simulink model "kalman_test"  (R2016b)
settings: Solver=VariableStepAuto  StartTime=0.0  StopTime=10  RelTol=1e-3
settings Model: Creator=Anass  LastModifiedBy=Anass

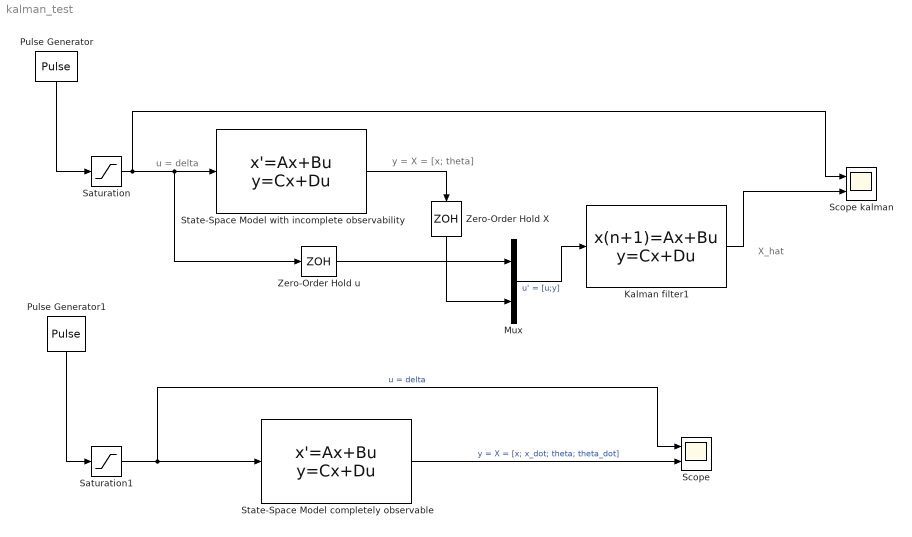
== system kalman_test ==
  note: X_hat
  note: y = X = [x; theta]
  note: u = delta
  Kalman filter1 : DiscreteStateSpace  A=|  B=|  C=eye(4)  D=zeros(4,3)  X0=[1;0;pi;0]  SampleTime=0.01  StateIdentifier=X_hat
      A=|
      | [    0.9697    0.0100   -0.0012         0;
      |    -0.0460    0.8959   -0.0171         0;
      |    -0.0012         0    0.9939    0.0100;
      |     0.0129   -0.0431   -0.3693    0.9938]
      B=|
      | [         0    0.0303    0.0012;
      |     0.5129    0.0460    0.0171;
      |          0    0.0012    0.0061;
      |     0.2102   -0.0129    0.0019]
  Mux : Mux  Inputs=2
  Pulse Generator : DiscretePulseGenerator  PulseType=Time based  Amplitude=0.9  Period=10  PulseWidth=3.4
  Pulse Generator1 : DiscretePulseGenerator  PulseType=Time based  Amplitude=0.9  Period=10  PulseWidth=3.4
  Saturation : Saturate  UpperLimit=0.9  LowerLimit=-0.8
  Saturation1 : Saturate  UpperLimit=0.9  LowerLimit=-0.8
  "Scope " : Scope  NumInputPorts=2
  Scope kalman : Scope  NumInputPorts=2
  State-Space Model completely observable : StateSpace  A=|  B=|  C=eye(4)  D=[0; 0;0;0]  X0=[1; 0; pi; 0.1]
      A=|
      | [0    1.0000         0         0;
      |          0  -10.4100         0         0;
      |          0         0         0    1.0000;
      |          0    -4.3111   -36.7400   -0.6249]
      B=|
      | [0;
      |    51.2860;
      |          0;
      |   21.0230]
  State-Space Model with incomplete observability : StateSpace  A=|  B=|  C=[1 0 0 0;0 0 1 0]  D=[0; 0]  X0=[1; 0; pi; 0.1]
      A=|
      | [0    1.0000         0         0;
      |          0  -10.4100         0         0;
      |          0         0         0    1.0000;
      |          0    -4.3111   -36.7400   -0.6249]
      B=|
      | [0;
      |    51.2860;
      |          0;
      |   21.0230]
  "Zero-Order Hold X " : ZeroOrderHold  SampleTime=0.01
  "Zero-Order Hold u " : ZeroOrderHold  SampleTime=0.01
  wires:
  Pulse Generator/1 -> Saturation/1
  Saturation1/1 -> "Scope "/1, State-Space Model completely observable/1  "u = delta"
  Pulse Generator1/1 -> Saturation1/1
  Saturation/1 -> Scope kalman/1, State-Space Model with incomplete observability/1, "Zero-Order Hold u "/1
  State-Space Model with incomplete observability/1 -> "Zero-Order Hold X "/1
  "Zero-Order Hold X "/1 -> Mux/2
  "Zero-Order Hold u "/1 -> Mux/1
  Mux/1 -> Kalman filter1/1  "u' = [u;y]"
  Kalman filter1/1 -> Scope kalman/2
  State-Space Model completely observable/1 -> "Scope "/2  "y = X = [x; x_dot; theta; theta_dot]"
